simulink model "M3_motor_load_gearbox"  (Simulink 10.2)
settings: Solver=ode4  StartTime=0.0  StopTime=0.1  FixedStep=T_s  RelTol=1e-3
undefined symbols (not defined in the file): A_v, b_eq, b_v, J_eq, k, L, N_opt, omega_v, R, theta_0, V_bar
settings Model: Creator=michelefocchi  LastModifiedBy=michelefocchi
settings DataIOCC: SaveFormat=Dataset  SignalLoggingSaveFormat=Dataset  ReturnWorkspaceOutputs=on
settings OptimizationCC: LifeSpan=auto
settings DebuggingCC: UnderspecifiedInitializationDetection=Simplified  MergeDetectMultiDrivingBlocksExec=error  FcnCallInpInsideContextMsg=error  SFUnexpectedBacktrackingDiag=error  SFNoUnconditionalDefaultTransitionDiag=error  SFExecutionAtInitializationDiag=warning  ArithmeticOperatorsInVariantConditions=error
settings HardwareCC: ProdBitPerPointer=64  ProdBitPerSizeT=64  ProdBitPerPtrDiffT=64  ProdLargestAtomicFloat=Float  ProdIntDivRoundTo=Zero  ProdEndianess=LittleEndian  ProdWordSize=64  ProdHWDeviceType=Intel->x86-64 (Windows64)
settings ModelReferenceCC: PropagateSignalLabelsOutOfModel=on
settings SFSimCC: SimUseLocalCustomCode=on  CustomCodeUndefinedFunction=FilterOut
settings RTWCC: RTWUseLocalCustomCode=on
settings CodeAppCC: StateflowObjectComments=off
settings GRTTargetCC: TargetLangStandard=C99 (ISO)  CombineOutputUpdateFcns=on  GRTInterface=off
settings ConfigComp: CovMetricSettings=dwe  CovSaveCumulativeToWorkspaceVar=off  CovSaveSingleToWorkspaceVar=off  CovExternalEMLEnable=on

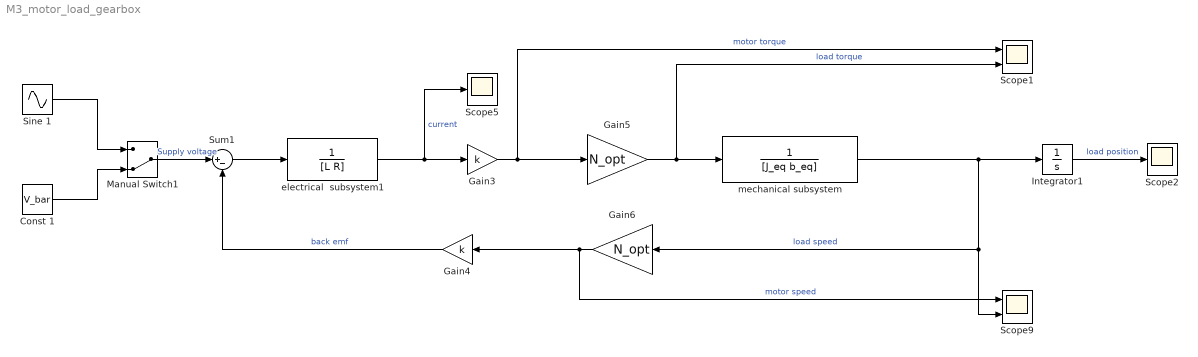
== system M3_motor_load_gearbox ==
  Const 1 : Constant  Value=V_bar
  Gain3 : Gain  Gain=k
  Gain4 : Gain  Gain=k
  Gain5 : Gain  Gain=N_opt
  Gain6 : Gain  Gain=N_opt
  Integrator1 : Integrator  InitialCondition=theta_0
  Manual Switch1 : ManualSwitch  CurrentSetting=0
  Scope1 : Scope  NumInputPorts=2
  Scope2 : Scope
  Scope5 : Scope
  Scope9 : Scope  NumInputPorts=2
  Sine 1 : Sin  Amplitude=A_v  Bias=b_v  Frequency=omega_v  SampleTime=0
  Sum1 : Sum  Inputs=|+-
  electrical  subsystem1 : TransferFcn  Denominator=[L R]
  mechanical subsystem : TransferFcn  Denominator=[J_eq b_eq]
  wires:
  Gain6/1 -> Scope9/1, Gain4/1  "motor speed"
  Gain4/1 -> Sum1/2  "back emf"
  electrical  subsystem1/1 -> Scope5/1, Gain3/1  "current"
  Manual Switch1/1 -> Sum1/1  "Supply voltage"
  Gain3/1 -> Scope1/1, Gain5/1  "motor torque"
  Integrator1/1 -> Scope2/1  "load position"
  Sine 1/1 -> Manual Switch1/1
  Gain5/1 -> Scope1/2, mechanical subsystem/1  "load torque"
  Sum1/1 -> electrical  subsystem1/1
  mechanical subsystem/1 -> Scope9/2, Gain6/1, Integrator1/1  "load speed"
  Const 1/1 -> Manual Switch1/2
